simulink model "lab_11_bdc3_target"  (R2021b)
settings: Solver=FixedStepDiscrete  StartTime=0.0  StopTime=inf  FixedStep=1e-4  RelTol=1e-3  EnableMultiTasking=on
libraries: speedgoatlib_IO102 x2, speedgoatlib_IO301 x2
settings Model: SimulationMode=external  Creator=tcraddoc  LastModifiedBy=wasynczu
settings SolverCC: ConcurrentTasks=on  AlgebraicLoopSolver=TrustRegion  PositivePriorityOrder=on
settings DataIOCC: SaveFormat=StructureWithTime  ReturnWorkspaceOutputs=off
settings OptimizationCC: BlockReduction=off  OptimizeBlockIOStorage=off  BufferReuse=off  GlobalBufferReuse=off  ExpressionFolding=off  LocalBlockOutputs=off
settings DebuggingCC: TasksWithSamePriorityMsg=none  SFMachineParentedDataDiag=warning  ArithmeticOperatorsInVariantConditions=warning
settings HardwareCC: ProdBitPerLong=64  ProdLongLongMode=on  ProdHWDeviceType=Intel->x86-64 (Linux 64)
settings SFSimCC: SimUseLocalCustomCode=off  CustomCodeUndefinedFunction=UseInterfaceOnly
settings RTWCC: Description=Simulink Real-Time  SystemTargetFile=slrealtime.tlc  TemplateMakefile=slrealtime_default_tmf  RTWUseLocalCustomCode=off  Toolchain=Simulink Real-Time Toolchain  BuildConfiguration=Faster Runs  CodeExecutionProfiling=on  TargetLang=C++
settings CodeAppCC: StateflowObjectComments=on

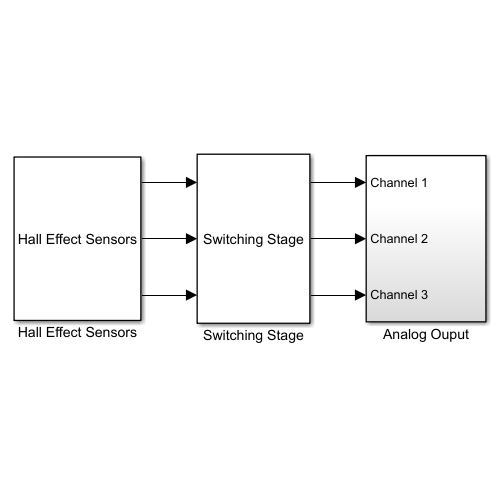
[thumbnail: Simulink's stored preview of the top-level diagram]
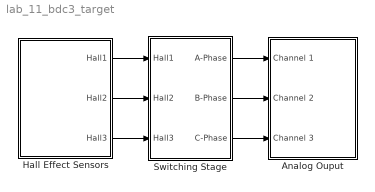
== system lab_11_bdc3_target ==
  Analog Ouput : Subsystem
  Hall Effect Sensors : Subsystem
      mask Display: disp('Hall Effect Sensors')
  Switching Stage : Subsystem
      mask Display: disp('Switching Stage')
  wires:
  Hall Effect Sensors/1(Hall1) -> Switching Stage/1(Hall1)
  Hall Effect Sensors/2(Hall2) -> Switching Stage/2(Hall2)
  Hall Effect Sensors/3(Hall3) -> Switching Stage/3(Hall3)
  Switching Stage/2(B-Phase) -> Analog Ouput/2(Channel 2)
  Switching Stage/1(A-Phase) -> Analog Ouput/1(Channel 1)
  Switching Stage/3(C-Phase) -> Analog Ouput/3(Channel 3)

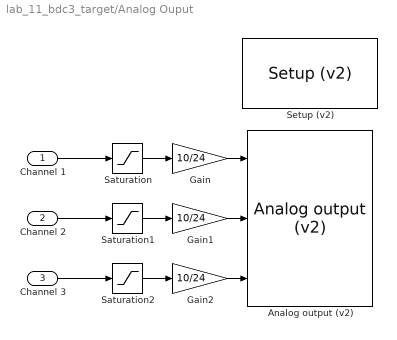
== system lab_11_bdc3_target/Analog Ouput ==
  Channel 1 : Inport
  Channel 2 : Inport  Port=2
  Channel 3 : Inport  Port=3
  "Analog output (v2) " : speedgoatlib_IO102/Analog output (v2)   id=1  channels=[1 2 3]  range=1  ts=1e-4  pciSlot=-1
      settings: SourceProductName=Simulink Real-Time: Speedgoat I/O Blockset
  Gain : Gain  Gain=10/24
  Gain1 : Gain  Gain=10/24
  Gain2 : Gain  Gain=10/24
  Saturation : Saturate  UpperLimit=24  LowerLimit=-24
  Saturation1 : Saturate  UpperLimit=24  LowerLimit=-24
  Saturation2 : Saturate  UpperLimit=24  LowerLimit=-24
  "Setup (v2) " : speedgoatlib_IO102/Setup (v2)   id=1  range=+-10V  cal=off  pciSlot=-1  adCoupling=Single-ended  adChannelMode=Multiple-channel (enter number of channels below)  adChannel=4  daChannel=[1,2,3]  daInitValue=[0]  daReset=[1]  DioDirectionLo=Input  DioDirectionHi=Output  doChannel=[9]  doInitValue=[0]  doReset=[1]  diChannel=[1]
      settings: SourceProductName=Simulink Real-Time: Speedgoat I/O Blockset
  wires:
  Saturation/1 -> Gain/1
  Saturation1/1 -> Gain1/1
  Saturation2/1 -> Gain2/1
  Gain1/1 -> "Analog output (v2) "/2
  Gain/1 -> "Analog output (v2) "/1
  Gain2/1 -> "Analog output (v2) "/3
  Channel 2/1 -> Saturation1/1
  Channel 3/1 -> Saturation2/1
  Channel 1/1 -> Saturation/1

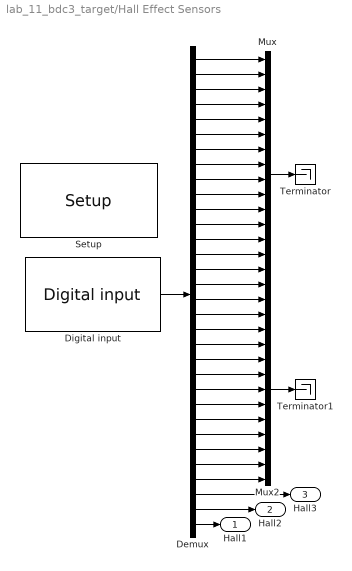
== system lab_11_bdc3_target/Hall Effect Sensors ==
  Demux : Demux  Outputs=32
  Digital input : speedgoatlib_IO301/DIO/Digital input  id=1  channelGroup=Upper  portType=1 port with 32 element vector of type boolean  lowerDirection=[1,1,1,1,1,0,0,0,0,0,0,0,1,0,0,0]  upperDirection=[1,1,1,1,1,1,1,1,0,0,0,0,0,0,0,0]  ts=1e-4  pciSlot=-1
      settings: SourceProductName=Simulink Real-Time: Speedgoat I/O Blockset
  Mux : Mux  Inputs=16
  Mux2 : Mux  Inputs=13
  Setup : speedgoatlib_IO301/Setup/Setup  group=Module setup  id=1  device_id=1  fpga1=speedgoat_IO301_default  pciSlot=-1  lowerDirection=[1, 1, 1, 1, 1, 0, 0, 0, 0, 0, 0, 0, 1, 0, 0, 0]  lowerReset=[1]  lowerValue=[0]  upperDirection=[1, 1, 1, 1, 1, 1, 1, 1, 0, 0, 0, 0, 0, 0, 0, 0]  upperReset=[1]  upperValue=[0]
      settings: SourceProductName=Simulink Real-Time: Speedgoat I/O Blockset
  Terminator : Terminator
  Terminator1 : Terminator
  Hall1 : Outport
  Hall2 : Outport  Port=2
  Hall3 : Outport  Port=3
  wires:
  Mux2/1 -> Terminator1/1
  Demux/16 -> Mux/16
  Demux/15 -> Mux/15
  Demux/14 -> Mux/14
  Demux/13 -> Mux/13
  Demux/12 -> Mux/12
  Demux/11 -> Mux/11
  Demux/10 -> Mux/10
  Demux/9 -> Mux/9
  Demux/8 -> Mux/8
  Demux/7 -> Mux/7
  Demux/6 -> Mux/6
  Demux/5 -> Mux/5
  Demux/4 -> Mux/4
  Demux/3 -> Mux/3
  Demux/2 -> Mux/2
  Demux/1 -> Mux/1
  Digital input/1 -> Demux/1
  Demux/17 -> Mux2/1
  Demux/18 -> Mux2/2
  Demux/19 -> Mux2/3
  Demux/20 -> Mux2/4
  Demux/21 -> Mux2/5
  Demux/22 -> Mux2/6
  Demux/23 -> Mux2/7
  Demux/24 -> Mux2/8
  Demux/25 -> Mux2/9
  Demux/26 -> Mux2/10
  Demux/27 -> Mux2/11
  Demux/28 -> Mux2/12
  Demux/29 -> Mux2/13
  Mux/1 -> Terminator/1
  Demux/30 -> Hall3/1
  Demux/31 -> Hall2/1
  Demux/32 -> Hall1/1

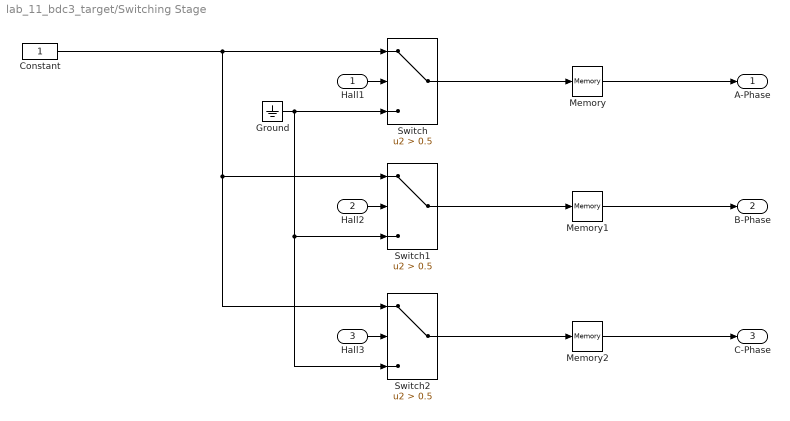
== system lab_11_bdc3_target/Switching Stage ==
  Hall1 : Inport
  Hall2 : Inport  Port=2
  Hall3 : Inport  Port=3
  Constant : Constant
  Ground : Ground
  Memory : Memory
  Memory1 : Memory
  Memory2 : Memory
  Switch : Switch  Criteria=u2 > Threshold  Threshold=0.5
  Switch1 : Switch  Criteria=u2 > Threshold  Threshold=0.5
  Switch2 : Switch  Criteria=u2 > Threshold  Threshold=0.5
  A-Phase : Outport
  B-Phase : Outport  Port=2
  C-Phase : Outport  Port=3
  wires:
  Hall1/1 -> Switch/2
  Ground/1 -> Switch2/3, Switch1/3, Switch/3
  Constant/1 -> Switch1/1, Switch2/1, Switch/1
  Hall2/1 -> Switch1/2
  Hall3/1 -> Switch2/2
  Memory/1 -> A-Phase/1
  Switch/1 -> Memory/1
  Memory1/1 -> B-Phase/1
  Switch1/1 -> Memory1/1
  Memory2/1 -> C-Phase/1
  Switch2/1 -> Memory2/1
